simulink model "BGOnly_5CH"  (R2017b)
settings: Solver=VariableStepAuto  StartTime=0.0  StopTime=60  RelTol=1e-3  EnableMultiTasking=on
values from neighbouring files (symbols this model uses):
  CHNoise = 1e-05    [Extension 1 Variables.mat]    (also in PlotChannelDiscrete.m = 1e-10; PlotChannelsExt.m = 0.0001; SelectivityFunction.m = 0.001)
  teta = 0.02    [Extension 1 Variables.mat]
  w_e = 0.9    [Extension 1 Variables.mat]    (also in PlotChannelsExt.m = 1)
  w_g = 1    [Extension 1 Variables.mat]
  w_minus = 1    [Extension 1 Variables.mat]    (also in PlotChannelsExt.m = 1.05)
  w_plus = 0.9    [Extension 1 Variables.mat]    (also in PlotChannelsExt.m = 1)
  w_s = 1    [Extension 1 Variables.mat]    (also in PlotChannelsExt.m)
  w_t = 0.9    [Extension 1 Variables.mat]    (also in PlotChannelsExt.m = 1)
undefined symbols (not defined in the file or in its folder): sigbuilder_block
libraries: fuzblock x25, simulink x8
settings Model: Creator=User  LastModifiedBy=acaso
settings DataIOCC: LimitDataPoints=on
settings OptimizationCC: LifeSpan=inf
settings DebuggingCC: AllowSymbolicDim=off  SFUnexpectedBacktrackingDiag=warning  SFNoUnconditionalDefaultTransitionDiag=warning  SFExecutionAtInitializationDiag=none
settings ModelReferenceCC: PropagateSignalLabelsOutOfModel=off
settings CodeAppCC: StateflowObjectComments=on
settings GRTTargetCC: TargetLangStandard=C89/C90 (ANSI)
settings ConfigComp: CovMetricSettings=dw  CovHtmlReporting=on  CovSaveCumulativeToWorkspaceVar=on  CovSaveSingleToWorkspaceVar=on  CovExternalEMLEnable=off

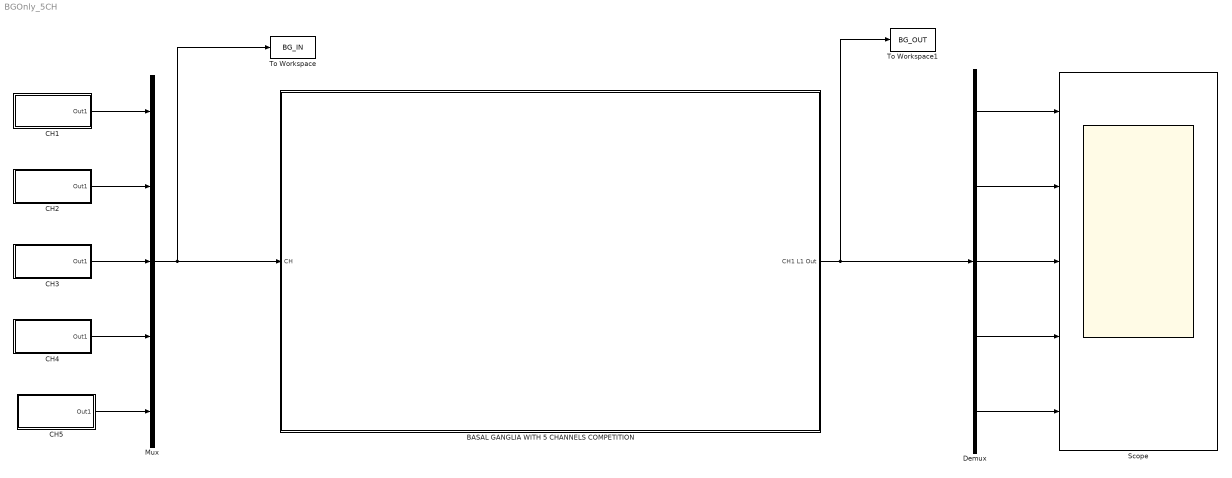
== system BGOnly_5CH ==
  BASAL GANGLIA WITH 5 CHANNELS COMPETITION : Subsystem
  "CH1 " : Subsystem
  CH2 : Subsystem
  "CH3 " : Subsystem
  "CH4 " : Subsystem
  "CH5 " : Subsystem
  Demux : Demux  Outputs=5
  Mux : Mux  Inputs=5
  Scope : Scope  NumInputPorts=5
  To Workspace : ToWorkspace  VariableName=BG_IN  SaveFormat=Timeseries  SampleTime=0.1
  To Workspace1 : ToWorkspace  VariableName=BG_OUT  SaveFormat=Timeseries  SampleTime=0.1
  wires:
  Mux/1 -> To Workspace/1, BASAL GANGLIA WITH 5 CHANNELS COMPETITION/1("CH ")
  BASAL GANGLIA WITH 5 CHANNELS COMPETITION/1(CH1 L1 Out) -> To Workspace1/1, Demux/1
  Demux/5 -> Scope/5
  Demux/4 -> Scope/4
  Demux/3 -> Scope/3
  Demux/2 -> Scope/2
  Demux/1 -> Scope/1
  "CH1 "/1(Out1) -> Mux/1
  CH2/1(Out1) -> Mux/2
  "CH3 "/1(Out1) -> Mux/3
  "CH4 "/1(Out1) -> Mux/4
  "CH5 "/1(Out1) -> Mux/5

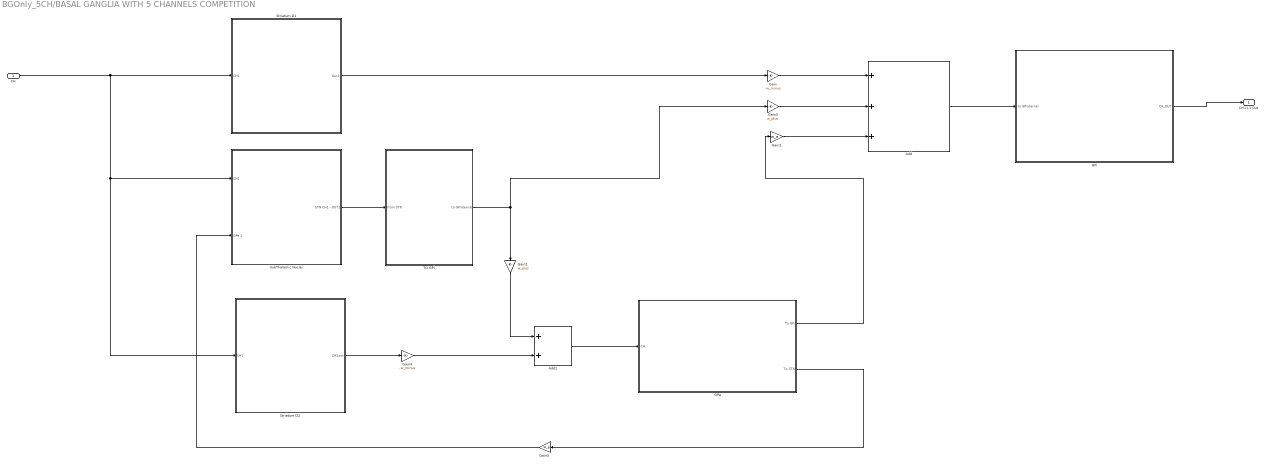
== system BGOnly_5CH/BASAL GANGLIA WITH 5 CHANNELS COMPETITION ==
  "CH " : Inport
  Add : Sum  Inputs=3
  Add1 : Sum  Inputs=2
  GPe : Subsystem  TreatAsAtomicUnit=on
  GPi : Subsystem
  Gain : Gain  Gain=-w_minus
  Gain1 : Gain  Gain=w_e
  Gain2 : Gain  Gain=w_plus
  Gain3 : Gain  Gain=w_plus
  Gain4 : Gain  Gain=-w_minus
  Gain5 : Gain  Gain=-w_g
  "Striatum D1 " : Subsystem
  Striatum D2 : Subsystem
  SubThalamic Nuclei : Subsystem
  TO GPi : Subsystem
  CH1 L1 Out : Outport
  wires:
  TO GPi/1(to GPinternal) -> Gain3/1, Gain2/1
  GPi/1("CH_OUT ") -> CH1 L1 Out/1
  "CH "/1 -> Striatum D2/1(CH1), SubThalamic Nuclei/1(CH1), "Striatum D1 "/1(CH1)
  "Striatum D1 "/1(Out1) -> Gain/1
  SubThalamic Nuclei/1(STN CH1 - OUT1) -> TO GPi/1("from STN ")
  GPe/1(To GPi) -> Gain1/1
  Gain/1 -> Add/1
  Gain3/1 -> Add/2
  Gain1/1 -> Add/3
  Striatum D2/1(CH1out) -> Gain4/1
  Gain2/1 -> Add1/1
  Gain4/1 -> Add1/2
  Add1/1 -> GPe/1(CH)
  GPe/2(To STN) -> Gain5/1
  Gain5/1 -> SubThalamic Nuclei/2(GPe 1)
  Add/1 -> GPi/1("to GPinternal ")

== system BGOnly_5CH/CH1  ==
  Add : Sum
  Band-Limited White Noise : simulink/Sources/Band-Limited White Noise  Cov=[CHNoise]  Ts=0.1  seed=[23341]
  "CHANNEL1 IN " : Subsystem  Tag=STV Subsys  LoadFcn=sigbuilder_block('load');  StartFcn=sigbuilder_block('start');  StopFcn=sigbuilder_block('stop');  ClipboardFcn=sigbuilder_block('clipboard');  mask(Sigbuilder block){tuvar=[0:10]}
      mask help: Simulink:masks:SigbuilderBlock_MD
      mask init:
      | if ~strcmp(get_param(bdroot(gcbh),'SimulationStatus'),'stopped') tuvar = sigbuilder_block('maskInit'); end
      settings: CopyFcn=sigbuilder_block('copy');  DeleteFcn=sigbuilder_block('delete');  ModelCloseFcn=sigbuilder_block('modelClose');  PreSaveFcn=sigbuilder_block('preSave');  PauseFcn=sigbuilder_block('pause');  ContinueFcn=sigbuilder_block('continue');  NameChangeFcn=sigbuilder_block('namechange');  OpenFcn=sigbuilder_block('open',[5.4 5.4 1141.2 580.8 ]);  CloseFcn=sigbuilder_block('close');
      mask Display: plot(0, 0, 100, 100,[2, 2, 32, 32, 2], [68, 8, 8, 68, 68],[32, 2], [38, 38], [32, 19, 2],[53, 60, 44], [32, 17, 17, 2],[16, 16, 31, 31]);txt = getActiveGroup(gcbh);text(2, 100, txt,'verticalAlignment', 'top');
  Out1 : Outport
  wires:
  Band-Limited White Noise/1 -> Add/2
  Add/1 -> Out1/1
  "CHANNEL1 IN "/1(Signal 1) -> Add/1

== system BGOnly_5CH/CH2 ==
  Add : Sum
  Band-Limited White Noise : simulink/Sources/Band-Limited White Noise  Cov=[CHNoise]  Ts=0.1  seed=[23341]
  "CHANNEL2 IN " : Subsystem  Tag=STV Subsys  LoadFcn=sigbuilder_block('load');  StartFcn=sigbuilder_block('start');  StopFcn=sigbuilder_block('stop');  ClipboardFcn=sigbuilder_block('clipboard');  mask(Sigbuilder block){tuvar=[0:10]}
      mask help: Simulink:masks:SigbuilderBlock_MD
      mask init:
      | if ~strcmp(get_param(bdroot(gcbh),'SimulationStatus'),'stopped') tuvar = sigbuilder_block('maskInit'); end
      settings: CopyFcn=sigbuilder_block('copy');  DeleteFcn=sigbuilder_block('delete');  ModelCloseFcn=sigbuilder_block('modelClose');  PreSaveFcn=sigbuilder_block('preSave');  PauseFcn=sigbuilder_block('pause');  ContinueFcn=sigbuilder_block('continue');  NameChangeFcn=sigbuilder_block('namechange');  OpenFcn=sigbuilder_block('open',[161.4 5.4 877.8 580.8 ]);  CloseFcn=sigbuilder_block('close');
      mask Display: plot(0, 0, 100, 100,[2, 2, 32, 32, 2], [68, 8, 8, 68, 68],[32, 2], [38, 38], [32, 19, 2],[53, 60, 44], [32, 17, 17, 2],[16, 16, 31, 31]);txt = getActiveGroup(gcbh);text(2, 100, txt,'verticalAlignment', 'top');
  Out1 : Outport
  wires:
  Band-Limited White Noise/1 -> Add/2
  Add/1 -> Out1/1
  "CHANNEL2 IN "/3(Signal 3) -> Add/1

== system BGOnly_5CH/CH3  ==
  Add : Sum
  Band-Limited White Noise : simulink/Sources/Band-Limited White Noise  Cov=[CHNoise]  Ts=0.1  seed=[23341]
  "CHANNEL2 IN " : Subsystem  Tag=STV Subsys  LoadFcn=sigbuilder_block('load');  StartFcn=sigbuilder_block('start');  StopFcn=sigbuilder_block('stop');  ClipboardFcn=sigbuilder_block('clipboard');  mask(Sigbuilder block){tuvar=[0:10]}
      mask help: Simulink:masks:SigbuilderBlock_MD
      mask init:
      | if ~strcmp(get_param(bdroot(gcbh),'SimulationStatus'),'stopped') tuvar = sigbuilder_block('maskInit'); end
      settings: CopyFcn=sigbuilder_block('copy');  DeleteFcn=sigbuilder_block('delete');  ModelCloseFcn=sigbuilder_block('modelClose');  PreSaveFcn=sigbuilder_block('preSave');  PauseFcn=sigbuilder_block('pause');  ContinueFcn=sigbuilder_block('continue');  NameChangeFcn=sigbuilder_block('namechange');  OpenFcn=sigbuilder_block('open',[5.4 5.4 1141.2 580.8 ]);  CloseFcn=sigbuilder_block('close');
      mask Display: plot(0, 0, 100, 100,[2, 2, 32, 32, 2], [68, 8, 8, 68, 68],[32, 2], [38, 38], [32, 19, 2],[53, 60, 44], [32, 17, 17, 2],[16, 16, 31, 31]);txt = getActiveGroup(gcbh);text(2, 100, txt,'verticalAlignment', 'top');
  Out1 : Outport
  wires:
  Band-Limited White Noise/1 -> Add/2
  Add/1 -> Out1/1
  "CHANNEL2 IN "/1(Signal 3) -> Add/1

== system BGOnly_5CH/CH4  ==
  Add : Sum
  Band-Limited White Noise : simulink/Sources/Band-Limited White Noise  Cov=[CHNoise]  Ts=0.1  seed=[23341]
  "CHANNEL2 IN " : Subsystem  Tag=STV Subsys  LoadFcn=sigbuilder_block('load');  StartFcn=sigbuilder_block('start');  StopFcn=sigbuilder_block('stop');  ClipboardFcn=sigbuilder_block('clipboard');  mask(Sigbuilder block){tuvar=[0:10]}
      mask help: Simulink:masks:SigbuilderBlock_MD
      mask init:
      | if ~strcmp(get_param(bdroot(gcbh),'SimulationStatus'),'stopped') tuvar = sigbuilder_block('maskInit'); end
      settings: CopyFcn=sigbuilder_block('copy');  DeleteFcn=sigbuilder_block('delete');  ModelCloseFcn=sigbuilder_block('modelClose');  PreSaveFcn=sigbuilder_block('preSave');  PauseFcn=sigbuilder_block('pause');  ContinueFcn=sigbuilder_block('continue');  NameChangeFcn=sigbuilder_block('namechange');  OpenFcn=sigbuilder_block('open',[5.4 5.4 1141.2 580.8 ]);  CloseFcn=sigbuilder_block('close');
      mask Display: plot(0, 0, 100, 100,[2, 2, 32, 32, 2], [68, 8, 8, 68, 68],[32, 2], [38, 38], [32, 19, 2],[53, 60, 44], [32, 17, 17, 2],[16, 16, 31, 31]);txt = getActiveGroup(gcbh);text(2, 100, txt,'verticalAlignment', 'top');
  Out1 : Outport
  wires:
  Band-Limited White Noise/1 -> Add/2
  Add/1 -> Out1/1
  "CHANNEL2 IN "/1(Signal 3) -> Add/1

== system BGOnly_5CH/CH5  ==
  Add : Sum
  Band-Limited White Noise : simulink/Sources/Band-Limited White Noise  Cov=[CHNoise]  Ts=0.1  seed=[23341]
  "CHANNEL2 IN " : Subsystem  Tag=STV Subsys  LoadFcn=sigbuilder_block('load');  StartFcn=sigbuilder_block('start');  StopFcn=sigbuilder_block('stop');  ClipboardFcn=sigbuilder_block('clipboard');  mask(Sigbuilder block){tuvar=[0:10]}
      mask help: Simulink:masks:SigbuilderBlock_MD
      mask init:
      | if ~strcmp(get_param(bdroot(gcbh),'SimulationStatus'),'stopped') tuvar = sigbuilder_block('maskInit'); end
      settings: CopyFcn=sigbuilder_block('copy');  DeleteFcn=sigbuilder_block('delete');  ModelCloseFcn=sigbuilder_block('modelClose');  PreSaveFcn=sigbuilder_block('preSave');  PauseFcn=sigbuilder_block('pause');  ContinueFcn=sigbuilder_block('continue');  NameChangeFcn=sigbuilder_block('namechange');  OpenFcn=sigbuilder_block('open',[5.4 5.4 1141.2 580.8 ]);  CloseFcn=sigbuilder_block('close');
      mask Display: plot(0, 0, 100, 100,[2, 2, 32, 32, 2], [68, 8, 8, 68, 68],[32, 2], [38, 38], [32, 19, 2],[53, 60, 44], [32, 17, 17, 2],[16, 16, 31, 31]);txt = getActiveGroup(gcbh);text(2, 100, txt,'verticalAlignment', 'top');
  Out1 : Outport
  wires:
  Band-Limited White Noise/1 -> Add/2
  Add/1 -> Out1/1
  "CHANNEL2 IN "/1(Signal 3) -> Add/1

== system BGOnly_5CH/BASAL GANGLIA WITH 5 CHANNELS COMPETITION/GPe ==
  CH : Inport
  GPe CH1 : Subsystem
  To GPi : Outport
  To STN : Outport  Port=2
  wires:
  CH/1 -> GPe CH1/1(In)
  GPe CH1/1(To GPi) -> To GPi/1
  GPe CH1/2(To STN) -> To STN/1

== system BGOnly_5CH/BASAL GANGLIA WITH 5 CHANNELS COMPETITION/GPi ==
  "to GPinternal " : Inport
  GPinternal : Subsystem
  "CH_OUT " : Outport
  wires:
  "to GPinternal "/1 -> GPinternal/1("to GPinternal ")
  GPinternal/1(To Thal) -> "CH_OUT "/1

== system BGOnly_5CH/BASAL GANGLIA WITH 5 CHANNELS COMPETITION/Striatum D1  ==
  CH1 : Inport
  "Striatum D1 " : Subsystem
  Out1 : Outport
  wires:
  CH1/1 -> "Striatum D1 "/1(Channel)
  "Striatum D1 "/1(Striatum D1 Out) -> Out1/1

== system BGOnly_5CH/BASAL GANGLIA WITH 5 CHANNELS COMPETITION/Striatum D2 ==
  CH1 : Inport
  Scope : Scope
  "Striatum D2 " : Subsystem
  CH1out : Outport
  wires:
  "Striatum D2 "/1(Striatum D1 Out) -> Scope/1, CH1out/1
  CH1/1 -> "Striatum D2 "/1(Channel)

== system BGOnly_5CH/BASAL GANGLIA WITH 5 CHANNELS COMPETITION/SubThalamic Nuclei ==
  CH1 : Inport
  GPe 1 : Inport  Port=2
  "SubThalamic Nucleus (STN) " : Subsystem
  STN CH1 - OUT1 : Outport
  wires:
  CH1/1 -> "SubThalamic Nucleus (STN) "/1(Channel)
  GPe 1/1 -> "SubThalamic Nucleus (STN) "/2(GPe Inp)
  "SubThalamic Nucleus (STN) "/1(STN Out1) -> STN CH1 - OUT1/1

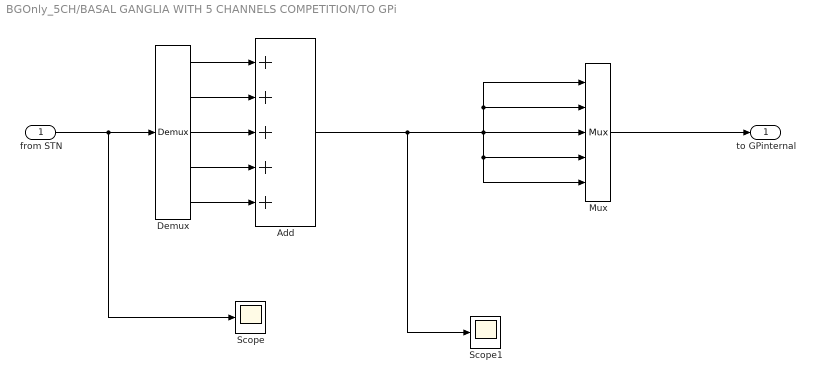
== system BGOnly_5CH/BASAL GANGLIA WITH 5 CHANNELS COMPETITION/TO GPi ==
  "from STN " : Inport
  Add : Sum  Inputs=5
  Demux : Demux  Outputs=5
  Mux : Mux  Inputs=5
  Scope : Scope
  Scope1 : Scope
  to GPinternal : Outport
  wires:
  "from STN "/1 -> Scope/1, Demux/1
  Demux/1 -> Add/1
  Demux/2 -> Add/2
  Demux/3 -> Add/3
  Demux/4 -> Add/4
  Demux/5 -> Add/5
  Add/1 -> Scope1/1, Mux/1, Mux/2, Mux/3, Mux/4, Mux/5
  Mux/1 -> to GPinternal/1

== system BGOnly_5CH/CH1 /CHANNEL1 IN  ==
  Demux : Demux  Tag=STV Demux  Outputs=2
  FromWs : FromWorkspace  Tag=STV FromWs  VariableName=tuvar  SampleTime=0
      SigBuilderData=|
      | common.afterFinalStr = 'Extrapolate'
      | common.sampleTime = 0
      | dataSet.timeRange = [0 35]
      | dataSet.name = 'Group 1'
      | sbobj.Groups.Name = 'Group 1'
      | sbobj.Groups.Signals(1).Name = 'Signal 1'
      | sbobj.Groups.Signals(1).XData = [0 0.125 0.25 0.375 0.5 0.625 0.75 0.875 1 1.125 1.25 1.375 1.5 1.625 1.75 1.875 2 2.125 2.25 2.375 2.5 2.625 2.75 2.875 3 3.125 3.25 3.375 3.5 3.625 3.75 3.875 4 4.125 4.25 4.375 4.5 4.625 4.75 4.875 5 5.125 5.25 5.375 5.5 5.625 5.75 5.875 6 6.125 6.25 6.375 6.5 6.625 6.75 6.875 7 7.125 7.25 7.375 7.5 7.625 7.75 7.875 8 8.125 8.25 8.375 8.5 8.625 8.75 8.875 9 9.125 9.25 9.375 9.5 9.625 9.75 9.875 10 10.125 10.25 10.375 10.5 10.625 10.75 10.875 11 11.125 11.25 11.375 11.5 11.625 11.75 11.875 12 12.125 12.25 12.375 12.5 12.625 12.75 12.875 13 13.125 13.25 13.375 13.5 13.625 13.75 13.875 14 14.125 14.25 14.375 14.5 14.625 14.75 14.875 15 15.125 15.25 15.375 15.5 15.625 15.75 15.875 16 16.125 16.25 16.375 16.5 16.625 16.75 16.875 17 17.125 17.25 17.375 17.5 17.625 17.75 17.875 18 18.125 18.25 18.375 18.5 18.625 18.75 18.875 19 19.125 19.25 19.375 19.5 19.625 19.75 19.875 20 20.125 20.25 20.375 20.5 20.625 20.75 20.875 21 21.125 21.25 21.375 21.5 21.625 21.75 21.875 22 22.125 22.25 22.375 22.5 22.625 22.75 22.875 23 23.125 23.25 23.375 23.5 23.625 23.75 23.875 24 24.125 24.25 24.375 24.5 24.625 24.75 24.875 25 25.125 25.25 25.375 25.5 25.625 25.75 25.875 26 26.125 26.25 26.375 26.5 26.625 26.75 26.875 27 27.125 27.25 27.375 27.5 27.625 27.75 27.875 28 28.125 28.25 28.375 28.5 28.625 28.75 28.875 29 29.125 29.25 29.375 29.5 29.625 29.75 29.875 30 30.125 30.25 30.375 30.5 30.625 30.75 30.875 31 31.125 31.25 31.375 31.5 31.625 31.75 31.875 32 32.125 32.25 32.375 32.5 32.625 32.75 32.875 33 33.125 33.25 33.375 33.5 33.625 33.75 33.875 34 34.125 34.25 34.375 34.5 34.625 34.75 34.875 35]
      | sbobj.Groups.Signals(1).YData = [1 1.70710678119 2 1.70710678119 1 0.292893218813 0 0.292893218813 1 1.70710678119 2 1.70710678119 ... (281 elements, 1x281)]
      | sbobj.Groups.Signals(2).Name = 'Signal 2'
      | sbobj.Groups.Signals(2).XData = [0 10 10 19.95 19.95 35]
      | sbobj.Groups.Signals(2).YData = [0 0 1 1 0 0]
      | sbobj.Groups.TimeRange = [0 35]
  Signal 1 : Outport  Tag=STV Outport
  Signal 2 : Outport  Tag=STV Outport  Port=2
  wires:
  Demux/1 -> Signal 1/1
  FromWs/1 -> Demux/1
  Demux/2 -> Signal 2/1

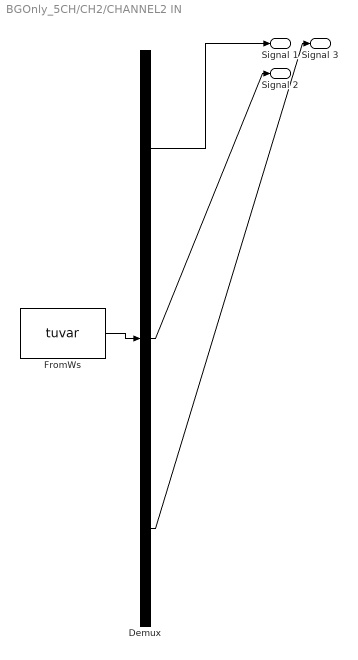
== system BGOnly_5CH/CH2/CHANNEL2 IN  ==
  Demux : Demux  Tag=STV Demux  Outputs=3
  FromWs : FromWorkspace  Tag=STV FromWs  VariableName=tuvar  SampleTime=0
      SigBuilderData=|
      | common.afterFinalStr = 'Extrapolate'
      | common.sampleTime = 0
      | dataSet.timeRange = [0 35]
      | dataSet.name = 'Group 1'
      | sbobj.Groups.Name = 'Group 1'
      | sbobj.Groups.Signals(1).Name = 'Signal 1'
      | sbobj.Groups.Signals(1).XData = [0 10 10 15.05 15.05 20 20 24.95 24.95 30 30 35]
      | sbobj.Groups.Signals(1).YData = [-0.002 -0.002 0.40108 0.402 0.598 0.598 0.898 0.898 0.405 0.405 -0.002 -0.002]
      | sbobj.Groups.Signals(2).Name = 'Signal 2'
      | sbobj.Groups.Signals(2).XData = [0 15 15 25.05 25.05 35]
      | sbobj.Groups.Signals(2).YData = [0 0 1 1 0 0]
      | sbobj.Groups.Signals(3).Name = 'Signal 3'
      | sbobj.Groups.Signals(3).XData = [0 0.25 0.5 0.75 1 1.25 1.5 1.75 2 2.25 2.5 2.75 3 3.25 3.5 3.75 4 4.25 4.5 4.75 5 5.25 5.5 5.75 6 6.25 6.5 6.75 7 7.25 7.5 7.75 8 8.25 8.5 8.75 9 9.25 9.5 9.75 10 10.25 10.5 10.75 11 11.25 11.5 11.75 12 12.25 12.5 12.75 13 13.25 13.5 13.75 14 14.25 14.5 14.75 15 15.25 15.5 15.75 16 16.25 16.5 16.75 17 17.25 17.5 17.75 18 18.25 18.5 18.75 19 19.25 19.5 19.75 20 20.25 20.5 20.75 21 21.25 21.5 21.75 22 22.25 22.5 22.75 23 23.25 23.5 23.75 24 24.25 24.5 24.75 25 25.25 25.5 25.75 26 26.25 26.5 26.75 27 27.25 27.5 27.75 28 28.25 28.5 28.75 29 29.25 29.5 29.75 30 30.25 30.5 30.75 31 31.25 31.5 31.75 32 32.25 32.5 32.75 33 33.25 33.5 33.75 34 34.25 34.5 34.75 35]
      | sbobj.Groups.Signals(3).YData = [1 1.70710678119 2 1.70710678119 1 0.292893218813 0 0.292893218813 1 1.70710678119 2 1.70710678119 1 0.292893218813 0 0.292893218813 1 1.70710678119 2 1.70710678119 1 0.292893218813 0 0.292893218813 1 1.70710678119 2 1.70710678119 1 0.292893218813 0 0.292893218813 1 1.70710678119 2 1.70710678119 1 0.292893218813 0 0.292893218813 1 1.70710678119 2 1.70710678119 1 0.292893218813 0 0.292893218813 1 1.70710678119 2 1.70710678119 1 0.292893218813 0 0.292893218813 1 1.70710678119 2 1.70710678119 1 0.292893218813 0 0.292893218813 1 1.70710678119 2 1.70710678119 1 0.292893218813 0 0.292893218813 1 1.70710678119 2 1.70710678119 1 0.292893218813 0 0.292893218813 1 1.70710678119 2 1.70710678119 1 0.292893218813 0 0.292893218813 1 1.70710678119 2 1.70710678119 1 0.292893218813 0 0.292893218813 1 1.70710678119 2 1.70710678119 1 0.292893218813 0 0.292893218813 1 1.70710678119 2 1.70710678119 1 0.292893218813 0 0.292893218813 1 1.70710678119 2 1.70710678119 1 0.292893218813 0 0.292893218813 1 1.70710678119 2 1.70710678119 1 0.292893218813 0 0.292893218813 1 1.70710678119 2 1.70710678119 1 0.292893218813 0 0.292893218813 1 1.70710678119 2 1.70710678119 1]
      | sbobj.Groups.TimeRange = [0 35]
  Signal 1 : Outport  Tag=STV Outport
  Signal 2 : Outport  Tag=STV Outport  Port=2
  Signal 3 : Outport  Tag=STV Outport  Port=3
  wires:
  Demux/1 -> Signal 1/1
  FromWs/1 -> Demux/1
  Demux/2 -> Signal 2/1
  Demux/3 -> Signal 3/1

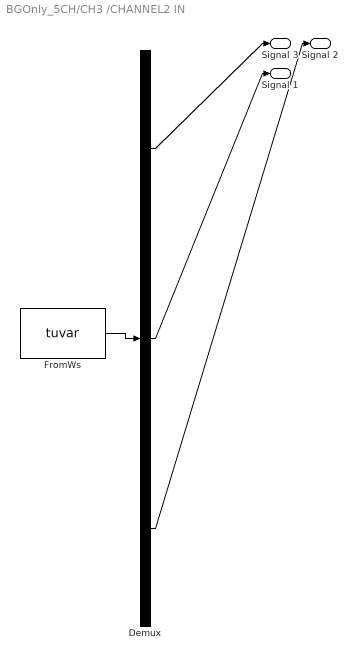
== system BGOnly_5CH/CH3 /CHANNEL2 IN  ==
  Demux : Demux  Tag=STV Demux  Outputs=3
  FromWs : FromWorkspace  Tag=STV FromWs  VariableName=tuvar  SampleTime=0
      SigBuilderData=|
      | common.afterFinalStr = 'Extrapolate'
      | common.sampleTime = 0
      | dataSet.timeRange = [0 35]
      | dataSet.name = 'Group 1'
      | sbobj.Groups.Name = 'Group 1'
      | sbobj.Groups.Signals(1).Name = 'Signal 3'
      | sbobj.Groups.Signals(1).XData = [0 35]
      | sbobj.Groups.Signals(1).YData = [0.195 0.195]
      | sbobj.Groups.Signals(2).Name = 'Signal 1'
      | sbobj.Groups.Signals(2).XData = [0 25 25 32.85 32.85 35]
      | sbobj.Groups.Signals(2).YData = [0 0 1 1 0 0]
      | sbobj.Groups.Signals(3).Name = 'Signal 2'
      | sbobj.Groups.Signals(3).XData = [0 0.5 1 1.5 2 2.5 3 3.5 4 4.5 5 5.5 6 6.5 7 7.5 8 8.5 9 9.5 10 10.5 11 11.5 12 12.5 13 13.5 14 14.5 15 15.5 16 16.5 17 17.5 18 18.5 19 19.5 20 20.5 21 21.5 22 22.5 23 23.5 24 24.5 25 25.5 26 26.5 27 27.5 28 28.5 29 29.5 30 30.5 31 31.5 32 32.5 33 33.5 34 34.5 35]
      | sbobj.Groups.Signals(3).YData = [1 1.70710678119 2 1.70710678119 1 0.292893218813 0 0.292893218813 1 1.70710678119 2 1.70710678119 1 0.292893218813 0 0.292893218813 1 1.70710678119 2 1.70710678119 1 0.292893218813 0 0.292893218813 1 1.70710678119 2 1.70710678119 1 0.292893218813 0 0.292893218813 1 1.70710678119 2 1.70710678119 1 0.292893218813 0 0.292893218813 1 1.70710678119 2 1.70710678119 1 0.292893218813 0 0.292893218813 1 1.70710678119 2 1.70710678119 1 0.292893218813 0 0.292893218813 1 1.70710678119 2 1.70710678119 1 0.292893218813 0 0.292893218813 1 1.70710678119 2 1.70710678119 1 0.292893218813 0]
      | sbobj.Groups.TimeRange = [0 35]
  Signal 3 : Outport  Tag=STV Outport
  Signal 1 : Outport  Tag=STV Outport  Port=2
  Signal 2 : Outport  Tag=STV Outport  Port=3
  wires:
  FromWs/1 -> Demux/1
  Demux/1 -> Signal 3/1
  Demux/2 -> Signal 1/1
  Demux/3 -> Signal 2/1

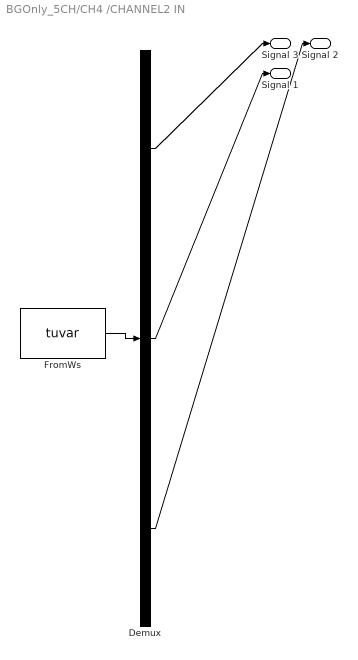
== system BGOnly_5CH/CH4 /CHANNEL2 IN  ==
  Demux : Demux  Tag=STV Demux  Outputs=3
  FromWs : FromWorkspace  Tag=STV FromWs  VariableName=tuvar  SampleTime=0
      SigBuilderData=|
      | common.afterFinalStr = 'Extrapolate'
      | common.sampleTime = 0
      | dataSet.timeRange = [0 35]
      | dataSet.name = 'Group 1'
      | sbobj.Groups.Name = 'Group 1'
      | sbobj.Groups.Signals(1).Name = 'Signal 3'
      | sbobj.Groups.Signals(1).XData = [0 35]
      | sbobj.Groups.Signals(1).YData = [0.12 0.12]
      | sbobj.Groups.Signals(2).Name = 'Signal 1'
      | sbobj.Groups.Signals(2).XData = [0 28.15 28.15 31.75 31.75 35]
      | sbobj.Groups.Signals(2).YData = [0 0 1 1 0 0]
      | sbobj.Groups.Signals(3).Name = 'Signal 2'
      | sbobj.Groups.Signals(3).XData = [0 1 2 3 4 5 6 7 8 9 10 11 12 13 14 15 16 17 18 19 20 21 22 23 24 25 26 27 28 29 30 31 32 33 34 35]
      | sbobj.Groups.Signals(3).YData = [1 1.70710678119 2 1.70710678119 1 0.292893218813 0 0.292893218813 1 1.70710678119 2 1.70710678119 1 0.292893218813 0 0.292893218813 1 1.70710678119 2 1.70710678119 1 0.292893218813 0 0.292893218813 1 1.70710678119 2 1.70710678119 1 0.292893218813 0 0.292893218813 1 1.70710678119 2 1.70710678119]
      | sbobj.Groups.TimeRange = [0 35]
  Signal 3 : Outport  Tag=STV Outport
  Signal 1 : Outport  Tag=STV Outport  Port=2
  Signal 2 : Outport  Tag=STV Outport  Port=3
  wires:
  FromWs/1 -> Demux/1
  Demux/1 -> Signal 3/1
  Demux/2 -> Signal 1/1
  Demux/3 -> Signal 2/1

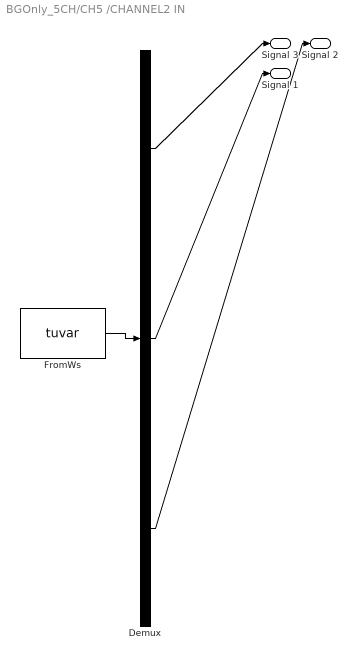
== system BGOnly_5CH/CH5 /CHANNEL2 IN  ==
  Demux : Demux  Tag=STV Demux  Outputs=3
  FromWs : FromWorkspace  Tag=STV FromWs  VariableName=tuvar  SampleTime=0
      SigBuilderData=|
      | common.afterFinalStr = 'Extrapolate'
      | common.sampleTime = 0
      | dataSet.timeRange = [0 35]
      | dataSet.name = 'Group 1'
      | sbobj.Groups.Name = 'Group 1'
      | sbobj.Groups.Signals(1).Name = 'Signal 3'
      | sbobj.Groups.Signals(1).XData = [0 35]
      | sbobj.Groups.Signals(1).YData = [0.085 0.085]
      | sbobj.Groups.Signals(2).Name = 'Signal 1'
      | sbobj.Groups.Signals(2).XData = [0 29.7 29.7 33.95 33.95 35]
      | sbobj.Groups.Signals(2).YData = [0.051 0.051 0.78 0.78 0.049 0.049]
      | sbobj.Groups.Signals(3).Name = 'Signal 2'
      | sbobj.Groups.Signals(3).XData = [0 2 4 6 8 10 12 14 16 18 20 22 24 26 28 30 32 34 35]
      | sbobj.Groups.Signals(3).YData = [1 1.70710678119 2 1.70710678119 1 0.292893218813 0 0.292893218813 1 1.70710678119 2 1.70710678119 1 0.292893218813 0 0.292893218813 1 1.70710678119 1.92387953251]
      | sbobj.Groups.TimeRange = [0 35]
  Signal 3 : Outport  Tag=STV Outport
  Signal 1 : Outport  Tag=STV Outport  Port=2
  Signal 2 : Outport  Tag=STV Outport  Port=3
  wires:
  FromWs/1 -> Demux/1
  Demux/1 -> Signal 3/1
  Demux/2 -> Signal 1/1
  Demux/3 -> Signal 2/1

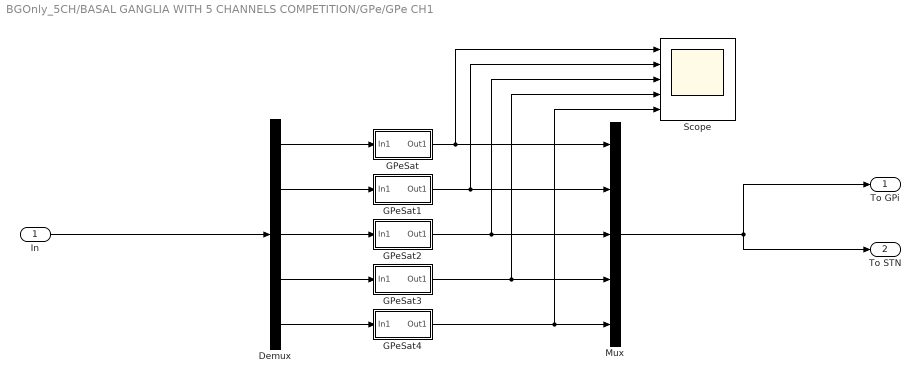
== system BGOnly_5CH/BASAL GANGLIA WITH 5 CHANNELS COMPETITION/GPe/GPe CH1 ==
  In : Inport
  Demux : Demux  Outputs=5
  GPeSat : Subsystem
  GPeSat1 : Subsystem
  GPeSat2 : Subsystem
  GPeSat3 : Subsystem
  GPeSat4 : Subsystem
  Mux : Mux  Inputs=5
  Scope : Scope  NumInputPorts=5
  To GPi : Outport
  To STN : Outport  Port=2
  wires:
  Mux/1 -> To STN/1, To GPi/1
  Demux/1 -> GPeSat/1(In1)
  GPeSat/1(Out1) -> Scope/1, Mux/1
  Demux/2 -> GPeSat1/1(In1)
  GPeSat1/1(Out1) -> Scope/2, Mux/2
  Demux/3 -> GPeSat2/1(In1)
  GPeSat2/1(Out1) -> Scope/3, Mux/3
  Demux/4 -> GPeSat3/1(In1)
  GPeSat3/1(Out1) -> Scope/4, Mux/4
  Demux/5 -> GPeSat4/1(In1)
  GPeSat4/1(Out1) -> Scope/5, Mux/5
  In/1 -> Demux/1

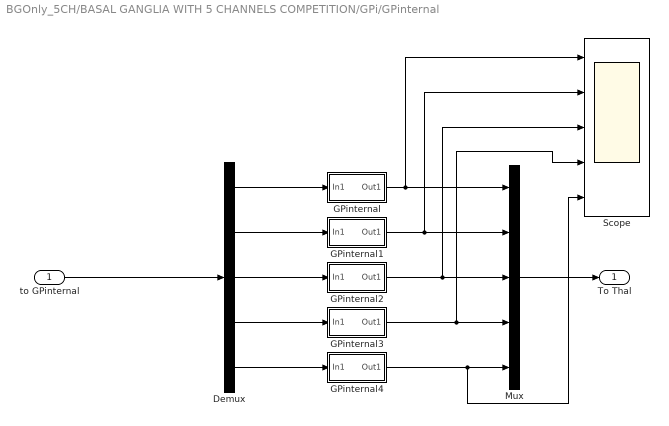
== system BGOnly_5CH/BASAL GANGLIA WITH 5 CHANNELS COMPETITION/GPi/GPinternal ==
  "to GPinternal " : Inport
  Demux : Demux  Outputs=5
  GPinternal : Subsystem
  GPinternal1 : Subsystem
  GPinternal2 : Subsystem
  GPinternal3 : Subsystem
  GPinternal4 : Subsystem
  Mux : Mux  Inputs=5
  Scope : Scope  NumInputPorts=5
  To Thal : Outport
  wires:
  Demux/1 -> GPinternal/1(In1)
  GPinternal/1(Out1) -> Mux/1, Scope/1
  Demux/2 -> GPinternal1/1(In1)
  Demux/3 -> GPinternal2/1(In1)
  GPinternal2/1(Out1) -> Scope/3, Mux/3
  Demux/4 -> GPinternal3/1(In1)
  GPinternal3/1(Out1) -> Scope/4, Mux/4
  Demux/5 -> GPinternal4/1(In1)
  GPinternal4/1(Out1) -> Scope/5, Mux/5
  Mux/1 -> To Thal/1
  GPinternal1/1(Out1) -> Scope/2, Mux/2
  "to GPinternal "/1 -> Demux/1

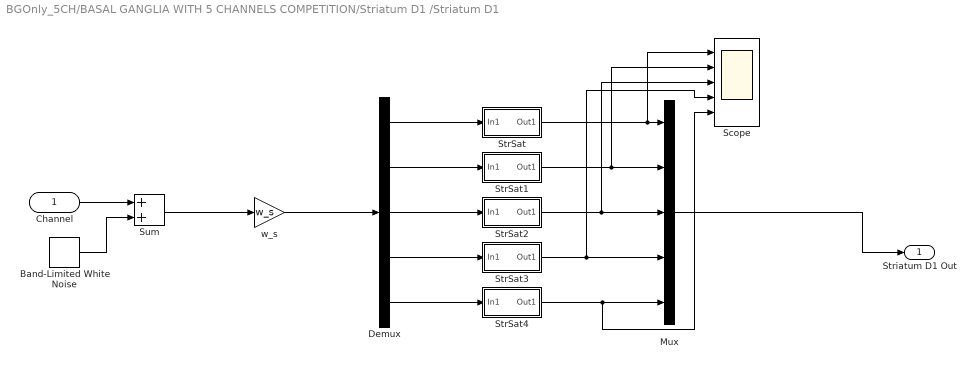
== system BGOnly_5CH/BASAL GANGLIA WITH 5 CHANNELS COMPETITION/Striatum D1 /Striatum D1  ==
  Channel : Inport
  Band-Limited White Noise : simulink/Sources/Band-Limited White Noise  Cov=[0]  Ts=0.1  seed=[23341]
  Demux : Demux  Outputs=5
  Mux : Mux  Inputs=5
  Scope : Scope  NumInputPorts=5
  StrSat : Subsystem
  StrSat1 : Subsystem
  StrSat2 : Subsystem
  StrSat3 : Subsystem
  StrSat4 : Subsystem
  Sum : Sum
  w_s : Gain  Gain=w_s
  Striatum D1 Out : Outport
  wires:
  Channel/1 -> Sum/1
  Sum/1 -> w_s/1
  Mux/1 -> Striatum D1 Out/1
  Band-Limited White Noise/1 -> Sum/2
  Demux/1 -> StrSat/1(In1)
  StrSat/1(Out1) -> Scope/1, Mux/1
  Demux/2 -> StrSat1/1(In1)
  StrSat1/1(Out1) -> Scope/2, Mux/2
  Demux/3 -> StrSat2/1(In1)
  StrSat2/1(Out1) -> Scope/3, Mux/3
  Demux/4 -> StrSat3/1(In1)
  StrSat3/1(Out1) -> Scope/4, Mux/4
  Demux/5 -> StrSat4/1(In1)
  StrSat4/1(Out1) -> Scope/5, Mux/5
  w_s/1 -> Demux/1

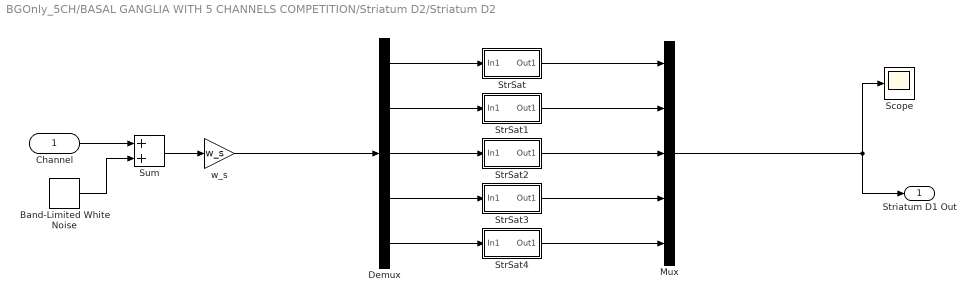
== system BGOnly_5CH/BASAL GANGLIA WITH 5 CHANNELS COMPETITION/Striatum D2/Striatum D2  ==
  Channel : Inport
  Band-Limited White Noise : simulink/Sources/Band-Limited White Noise  Cov=[0]  Ts=0.1  seed=[23341]
  Demux : Demux  Outputs=5
  Mux : Mux  Inputs=5
  Scope : Scope
  StrSat : Subsystem
  StrSat1 : Subsystem
  StrSat2 : Subsystem
  StrSat3 : Subsystem
  StrSat4 : Subsystem
  Sum : Sum
  w_s : Gain  Gain=w_s
  Striatum D1 Out : Outport
  wires:
  Channel/1 -> Sum/1
  Sum/1 -> w_s/1
  Mux/1 -> Striatum D1 Out/1, Scope/1
  Band-Limited White Noise/1 -> Sum/2
  Demux/1 -> StrSat/1(In1)
  StrSat/1(Out1) -> Mux/1
  Demux/2 -> StrSat1/1(In1)
  StrSat1/1(Out1) -> Mux/2
  Demux/3 -> StrSat2/1(In1)
  StrSat2/1(Out1) -> Mux/3
  Demux/4 -> StrSat3/1(In1)
  StrSat3/1(Out1) -> Mux/4
  Demux/5 -> StrSat4/1(In1)
  StrSat4/1(Out1) -> Mux/5
  w_s/1 -> Demux/1

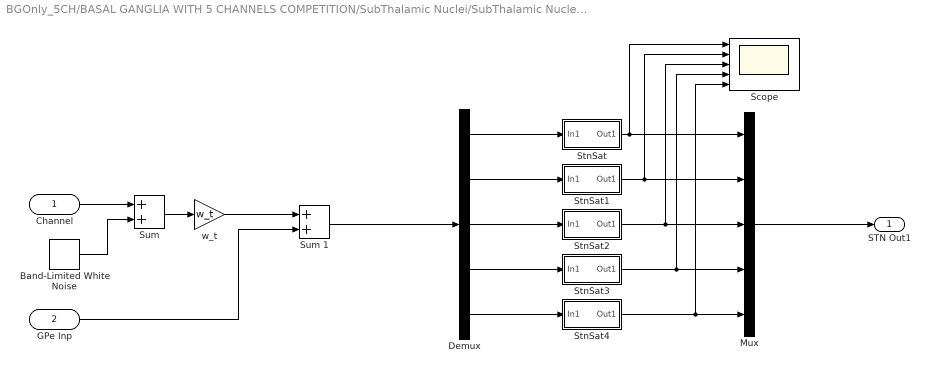
== system BGOnly_5CH/BASAL GANGLIA WITH 5 CHANNELS COMPETITION/SubThalamic Nuclei/SubThalamic Nucleus (STN)  ==
  Channel : Inport
  GPe Inp : Inport  Port=2
  Band-Limited White Noise : simulink/Sources/Band-Limited White Noise  Cov=[0]  Ts=0.1  seed=[23341]
  Demux : Demux  Outputs=5
  Mux : Mux  Inputs=5
  Scope : Scope  NumInputPorts=5
  StnSat : Subsystem
  StnSat1 : Subsystem
  StnSat2 : Subsystem
  StnSat3 : Subsystem
  StnSat4 : Subsystem
  "Sum " : Sum
  Sum 1 : Sum
  w_t : Gain  Gain=w_t
  STN Out1 : Outport
  wires:
  w_t/1 -> Sum 1/1
  Channel/1 -> "Sum "/1
  Band-Limited White Noise/1 -> "Sum "/2
  "Sum "/1 -> w_t/1
  GPe Inp/1 -> Sum 1/2
  Mux/1 -> STN Out1/1
  Demux/1 -> StnSat/1(In1)
  Demux/2 -> StnSat1/1(In1)
  StnSat1/1(Out1) -> Scope/2, Mux/2
  Demux/3 -> StnSat2/1(In1)
  StnSat2/1(Out1) -> Scope/3, Mux/3
  Demux/4 -> StnSat3/1(In1)
  StnSat3/1(Out1) -> Scope/4, Mux/4
  Demux/5 -> StnSat4/1(In1)
  StnSat4/1(Out1) -> Scope/5, Mux/5
  StnSat/1(Out1) -> Scope/1, Mux/1
  Sum 1/1 -> Demux/1

== system BGOnly_5CH/BASAL GANGLIA WITH 5 CHANNELS COMPETITION/GPe/GPe CH1/GPeSat ==
  In1 : Inport
  "Leaky-Integrator Striatum D1 " : ZeroPole  Zeros=[]  Poles=[-1/teta]  Gain=[1.5/teta]
  Sigmoidal MF : fuzblock/Membership  Functions/Sigmoidal MF  a=alpha_gpe  c=beta_gpe
      settings: SourceProductName=Fuzzy Logic Toolbox  SourceProductBaseCode=FL
  Out1 : Outport
  wires:
  Sigmoidal MF/1 -> Out1/1
  "Leaky-Integrator Striatum D1 "/1 -> Sigmoidal MF/1
  In1/1 -> "Leaky-Integrator Striatum D1 "/1

== system BGOnly_5CH/BASAL GANGLIA WITH 5 CHANNELS COMPETITION/GPe/GPe CH1/GPeSat1 ==
  In1 : Inport
  "Leaky-Integrator Striatum D1 " : ZeroPole  Zeros=[]  Poles=[-1/teta]  Gain=[1.5/teta]
  Sigmoidal MF : fuzblock/Membership  Functions/Sigmoidal MF  a=alpha_gpe  c=beta_gpe
      settings: SourceProductName=Fuzzy Logic Toolbox  SourceProductBaseCode=FL
  Out1 : Outport
  wires:
  Sigmoidal MF/1 -> Out1/1
  "Leaky-Integrator Striatum D1 "/1 -> Sigmoidal MF/1
  In1/1 -> "Leaky-Integrator Striatum D1 "/1

== system BGOnly_5CH/BASAL GANGLIA WITH 5 CHANNELS COMPETITION/GPe/GPe CH1/GPeSat2 ==
  In1 : Inport
  "Leaky-Integrator Striatum D1 " : ZeroPole  Zeros=[]  Poles=[-1/teta]  Gain=[1.5/teta]
  Sigmoidal MF : fuzblock/Membership  Functions/Sigmoidal MF  a=alpha_gpe  c=beta_gpe
      settings: SourceProductName=Fuzzy Logic Toolbox  SourceProductBaseCode=FL
  Out1 : Outport
  wires:
  Sigmoidal MF/1 -> Out1/1
  "Leaky-Integrator Striatum D1 "/1 -> Sigmoidal MF/1
  In1/1 -> "Leaky-Integrator Striatum D1 "/1

== system BGOnly_5CH/BASAL GANGLIA WITH 5 CHANNELS COMPETITION/GPe/GPe CH1/GPeSat3 ==
  In1 : Inport
  "Leaky-Integrator Striatum D1 " : ZeroPole  Zeros=[]  Poles=[-1/teta]  Gain=[1.5/teta]
  Sigmoidal MF : fuzblock/Membership  Functions/Sigmoidal MF  a=alpha_gpe  c=beta_gpe
      settings: SourceProductName=Fuzzy Logic Toolbox  SourceProductBaseCode=FL
  Out1 : Outport
  wires:
  Sigmoidal MF/1 -> Out1/1
  "Leaky-Integrator Striatum D1 "/1 -> Sigmoidal MF/1
  In1/1 -> "Leaky-Integrator Striatum D1 "/1

== system BGOnly_5CH/BASAL GANGLIA WITH 5 CHANNELS COMPETITION/GPe/GPe CH1/GPeSat4 ==
  In1 : Inport
  "Leaky-Integrator Striatum D1 " : ZeroPole  Zeros=[]  Poles=[-1/teta]  Gain=[1.5/teta]
  Sigmoidal MF : fuzblock/Membership  Functions/Sigmoidal MF  a=alpha_gpe  c=beta_gpe
      settings: SourceProductName=Fuzzy Logic Toolbox  SourceProductBaseCode=FL
  Out1 : Outport
  wires:
  Sigmoidal MF/1 -> Out1/1
  "Leaky-Integrator Striatum D1 "/1 -> Sigmoidal MF/1
  In1/1 -> "Leaky-Integrator Striatum D1 "/1

== system BGOnly_5CH/BASAL GANGLIA WITH 5 CHANNELS COMPETITION/GPi/GPinternal/GPinternal ==
  In1 : Inport
  "Leaky-Integrator Striatum D1 " : ZeroPole  Zeros=[]  Poles=[-1/teta]  Gain=[1.5/teta]
  Sigmoidal MF : fuzblock/Membership  Functions/Sigmoidal MF  a=alpha_gpi  c=beta_gpi
      settings: SourceProductName=Fuzzy Logic Toolbox  SourceProductBaseCode=FL
  Out1 : Outport
  wires:
  Sigmoidal MF/1 -> Out1/1
  "Leaky-Integrator Striatum D1 "/1 -> Sigmoidal MF/1
  In1/1 -> "Leaky-Integrator Striatum D1 "/1

== system BGOnly_5CH/BASAL GANGLIA WITH 5 CHANNELS COMPETITION/GPi/GPinternal/GPinternal1 ==
  In1 : Inport
  "Leaky-Integrator Striatum D1 " : ZeroPole  Zeros=[]  Poles=[-1/teta]  Gain=[1.5/teta]
  Sigmoidal MF : fuzblock/Membership  Functions/Sigmoidal MF  a=alpha_gpi  c=beta_gpi
      settings: SourceProductName=Fuzzy Logic Toolbox  SourceProductBaseCode=FL
  Out1 : Outport
  wires:
  Sigmoidal MF/1 -> Out1/1
  "Leaky-Integrator Striatum D1 "/1 -> Sigmoidal MF/1
  In1/1 -> "Leaky-Integrator Striatum D1 "/1

== system BGOnly_5CH/BASAL GANGLIA WITH 5 CHANNELS COMPETITION/GPi/GPinternal/GPinternal2 ==
  In1 : Inport
  "Leaky-Integrator Striatum D1 " : ZeroPole  Zeros=[]  Poles=[-1/teta]  Gain=[1.5/teta]
  Sigmoidal MF : fuzblock/Membership  Functions/Sigmoidal MF  a=alpha_gpi  c=beta_gpi
      settings: SourceProductName=Fuzzy Logic Toolbox  SourceProductBaseCode=FL
  Out1 : Outport
  wires:
  Sigmoidal MF/1 -> Out1/1
  "Leaky-Integrator Striatum D1 "/1 -> Sigmoidal MF/1
  In1/1 -> "Leaky-Integrator Striatum D1 "/1

== system BGOnly_5CH/BASAL GANGLIA WITH 5 CHANNELS COMPETITION/GPi/GPinternal/GPinternal3 ==
  In1 : Inport
  "Leaky-Integrator Striatum D1 " : ZeroPole  Zeros=[]  Poles=[-1/teta]  Gain=[1.5/teta]
  Sigmoidal MF : fuzblock/Membership  Functions/Sigmoidal MF  a=alpha_gpi  c=beta_gpi
      settings: SourceProductName=Fuzzy Logic Toolbox  SourceProductBaseCode=FL
  Out1 : Outport
  wires:
  Sigmoidal MF/1 -> Out1/1
  "Leaky-Integrator Striatum D1 "/1 -> Sigmoidal MF/1
  In1/1 -> "Leaky-Integrator Striatum D1 "/1

== system BGOnly_5CH/BASAL GANGLIA WITH 5 CHANNELS COMPETITION/GPi/GPinternal/GPinternal4 ==
  In1 : Inport
  "Leaky-Integrator Striatum D1 " : ZeroPole  Zeros=[]  Poles=[-1/teta]  Gain=[1.5/teta]
  Sigmoidal MF : fuzblock/Membership  Functions/Sigmoidal MF  a=alpha_gpi  c=beta_gpi
      settings: SourceProductName=Fuzzy Logic Toolbox  SourceProductBaseCode=FL
  Out1 : Outport
  wires:
  Sigmoidal MF/1 -> Out1/1
  "Leaky-Integrator Striatum D1 "/1 -> Sigmoidal MF/1
  In1/1 -> "Leaky-Integrator Striatum D1 "/1

== system BGOnly_5CH/BASAL GANGLIA WITH 5 CHANNELS COMPETITION/Striatum D1 /Striatum D1 /StrSat ==
  In1 : Inport
  "Leaky-Integrator Striatum D1 " : ZeroPole  Zeros=[]  Poles=[-1/teta]  Gain=[1.5/teta]
  Sigmoidal MF : fuzblock/Membership  Functions/Sigmoidal MF  a=alpha_str  c=beta_str
      settings: SourceProductName=Fuzzy Logic Toolbox  SourceProductBaseCode=FL
  Out1 : Outport
  wires:
  Sigmoidal MF/1 -> Out1/1
  "Leaky-Integrator Striatum D1 "/1 -> Sigmoidal MF/1
  In1/1 -> "Leaky-Integrator Striatum D1 "/1

== system BGOnly_5CH/BASAL GANGLIA WITH 5 CHANNELS COMPETITION/Striatum D1 /Striatum D1 /StrSat1 ==
  In1 : Inport
  "Leaky-Integrator Striatum D1 " : ZeroPole  Zeros=[]  Poles=[-1/teta]  Gain=[1.5/teta]
  Sigmoidal MF : fuzblock/Membership  Functions/Sigmoidal MF  a=alpha_str  c=beta_str
      settings: SourceProductName=Fuzzy Logic Toolbox  SourceProductBaseCode=FL
  Out1 : Outport
  wires:
  Sigmoidal MF/1 -> Out1/1
  "Leaky-Integrator Striatum D1 "/1 -> Sigmoidal MF/1
  In1/1 -> "Leaky-Integrator Striatum D1 "/1

== system BGOnly_5CH/BASAL GANGLIA WITH 5 CHANNELS COMPETITION/Striatum D1 /Striatum D1 /StrSat2 ==
  In1 : Inport
  "Leaky-Integrator Striatum D1 " : ZeroPole  Zeros=[]  Poles=[-1/teta]  Gain=[1.5/teta]
  Sigmoidal MF : fuzblock/Membership  Functions/Sigmoidal MF  a=alpha_str  c=beta_str
      settings: SourceProductName=Fuzzy Logic Toolbox  SourceProductBaseCode=FL
  Out1 : Outport
  wires:
  Sigmoidal MF/1 -> Out1/1
  "Leaky-Integrator Striatum D1 "/1 -> Sigmoidal MF/1
  In1/1 -> "Leaky-Integrator Striatum D1 "/1

== system BGOnly_5CH/BASAL GANGLIA WITH 5 CHANNELS COMPETITION/Striatum D1 /Striatum D1 /StrSat3 ==
  In1 : Inport
  "Leaky-Integrator Striatum D1 " : ZeroPole  Zeros=[]  Poles=[-1/teta]  Gain=[1.5/teta]
  Sigmoidal MF : fuzblock/Membership  Functions/Sigmoidal MF  a=alpha_str  c=beta_str
      settings: SourceProductName=Fuzzy Logic Toolbox  SourceProductBaseCode=FL
  Out1 : Outport
  wires:
  Sigmoidal MF/1 -> Out1/1
  "Leaky-Integrator Striatum D1 "/1 -> Sigmoidal MF/1
  In1/1 -> "Leaky-Integrator Striatum D1 "/1

== system BGOnly_5CH/BASAL GANGLIA WITH 5 CHANNELS COMPETITION/Striatum D1 /Striatum D1 /StrSat4 ==
  In1 : Inport
  "Leaky-Integrator Striatum D1 " : ZeroPole  Zeros=[]  Poles=[-1/teta]  Gain=[1.5/teta]
  Sigmoidal MF : fuzblock/Membership  Functions/Sigmoidal MF  a=alpha_str  c=beta_str
      settings: SourceProductName=Fuzzy Logic Toolbox  SourceProductBaseCode=FL
  Out1 : Outport
  wires:
  Sigmoidal MF/1 -> Out1/1
  "Leaky-Integrator Striatum D1 "/1 -> Sigmoidal MF/1
  In1/1 -> "Leaky-Integrator Striatum D1 "/1

== system BGOnly_5CH/BASAL GANGLIA WITH 5 CHANNELS COMPETITION/Striatum D2/Striatum D2 /StrSat ==
  In1 : Inport
  "Leaky-Integrator Striatum D1 " : ZeroPole  Zeros=[]  Poles=[-1/teta]  Gain=[1.5/teta]
  Sigmoidal MF : fuzblock/Membership  Functions/Sigmoidal MF  a=alpha_str  c=beta_str
      settings: SourceProductName=Fuzzy Logic Toolbox  SourceProductBaseCode=FL
  Out1 : Outport
  wires:
  Sigmoidal MF/1 -> Out1/1
  "Leaky-Integrator Striatum D1 "/1 -> Sigmoidal MF/1
  In1/1 -> "Leaky-Integrator Striatum D1 "/1

== system BGOnly_5CH/BASAL GANGLIA WITH 5 CHANNELS COMPETITION/Striatum D2/Striatum D2 /StrSat1 ==
  In1 : Inport
  "Leaky-Integrator Striatum D1 " : ZeroPole  Zeros=[]  Poles=[-1/teta]  Gain=[1.5/teta]
  Sigmoidal MF : fuzblock/Membership  Functions/Sigmoidal MF  a=alpha_str  c=beta_str
      settings: SourceProductName=Fuzzy Logic Toolbox  SourceProductBaseCode=FL
  Out1 : Outport
  wires:
  Sigmoidal MF/1 -> Out1/1
  "Leaky-Integrator Striatum D1 "/1 -> Sigmoidal MF/1
  In1/1 -> "Leaky-Integrator Striatum D1 "/1

== system BGOnly_5CH/BASAL GANGLIA WITH 5 CHANNELS COMPETITION/Striatum D2/Striatum D2 /StrSat2 ==
  In1 : Inport
  "Leaky-Integrator Striatum D1 " : ZeroPole  Zeros=[]  Poles=[-1/teta]  Gain=[1.5/teta]
  Sigmoidal MF : fuzblock/Membership  Functions/Sigmoidal MF  a=alpha_str  c=beta_str
      settings: SourceProductName=Fuzzy Logic Toolbox  SourceProductBaseCode=FL
  Out1 : Outport
  wires:
  Sigmoidal MF/1 -> Out1/1
  "Leaky-Integrator Striatum D1 "/1 -> Sigmoidal MF/1
  In1/1 -> "Leaky-Integrator Striatum D1 "/1

== system BGOnly_5CH/BASAL GANGLIA WITH 5 CHANNELS COMPETITION/Striatum D2/Striatum D2 /StrSat3 ==
  In1 : Inport
  "Leaky-Integrator Striatum D1 " : ZeroPole  Zeros=[]  Poles=[-1/teta]  Gain=[1.5/teta]
  Sigmoidal MF : fuzblock/Membership  Functions/Sigmoidal MF  a=alpha_str  c=beta_str
      settings: SourceProductName=Fuzzy Logic Toolbox  SourceProductBaseCode=FL
  Out1 : Outport
  wires:
  Sigmoidal MF/1 -> Out1/1
  "Leaky-Integrator Striatum D1 "/1 -> Sigmoidal MF/1
  In1/1 -> "Leaky-Integrator Striatum D1 "/1

== system BGOnly_5CH/BASAL GANGLIA WITH 5 CHANNELS COMPETITION/Striatum D2/Striatum D2 /StrSat4 ==
  In1 : Inport
  "Leaky-Integrator Striatum D1 " : ZeroPole  Zeros=[]  Poles=[-1/teta]  Gain=[1.5/teta]
  Sigmoidal MF : fuzblock/Membership  Functions/Sigmoidal MF  a=alpha_str  c=beta_str
      settings: SourceProductName=Fuzzy Logic Toolbox  SourceProductBaseCode=FL
  Out1 : Outport
  wires:
  Sigmoidal MF/1 -> Out1/1
  "Leaky-Integrator Striatum D1 "/1 -> Sigmoidal MF/1
  In1/1 -> "Leaky-Integrator Striatum D1 "/1

== system BGOnly_5CH/BASAL GANGLIA WITH 5 CHANNELS COMPETITION/SubThalamic Nuclei/SubThalamic Nucleus (STN) /StnSat ==
  In1 : Inport
  "Leaky-Integrator Striatum D1 " : ZeroPole  Zeros=[]  Poles=[-1/teta]  Gain=[1.5/teta]
  Sigmoidal MF : fuzblock/Membership  Functions/Sigmoidal MF  a=alpha_stn  c=beta_stn
      settings: SourceProductName=Fuzzy Logic Toolbox  SourceProductBaseCode=FL
  Out1 : Outport
  wires:
  Sigmoidal MF/1 -> Out1/1
  "Leaky-Integrator Striatum D1 "/1 -> Sigmoidal MF/1
  In1/1 -> "Leaky-Integrator Striatum D1 "/1

== system BGOnly_5CH/BASAL GANGLIA WITH 5 CHANNELS COMPETITION/SubThalamic Nuclei/SubThalamic Nucleus (STN) /StnSat1 ==
  In1 : Inport
  "Leaky-Integrator Striatum D1 " : ZeroPole  Zeros=[]  Poles=[-1/teta]  Gain=[1.5/teta]
  Sigmoidal MF : fuzblock/Membership  Functions/Sigmoidal MF  a=alpha_stn  c=beta_stn
      settings: SourceProductName=Fuzzy Logic Toolbox  SourceProductBaseCode=FL
  Out1 : Outport
  wires:
  Sigmoidal MF/1 -> Out1/1
  "Leaky-Integrator Striatum D1 "/1 -> Sigmoidal MF/1
  In1/1 -> "Leaky-Integrator Striatum D1 "/1

== system BGOnly_5CH/BASAL GANGLIA WITH 5 CHANNELS COMPETITION/SubThalamic Nuclei/SubThalamic Nucleus (STN) /StnSat2 ==
  In1 : Inport
  "Leaky-Integrator Striatum D1 " : ZeroPole  Zeros=[]  Poles=[-1/teta]  Gain=[1.5/teta]
  Sigmoidal MF : fuzblock/Membership  Functions/Sigmoidal MF  a=alpha_stn  c=beta_stn
      settings: SourceProductName=Fuzzy Logic Toolbox  SourceProductBaseCode=FL
  Out1 : Outport
  wires:
  Sigmoidal MF/1 -> Out1/1
  "Leaky-Integrator Striatum D1 "/1 -> Sigmoidal MF/1
  In1/1 -> "Leaky-Integrator Striatum D1 "/1

== system BGOnly_5CH/BASAL GANGLIA WITH 5 CHANNELS COMPETITION/SubThalamic Nuclei/SubThalamic Nucleus (STN) /StnSat3 ==
  In1 : Inport
  "Leaky-Integrator Striatum D1 " : ZeroPole  Zeros=[]  Poles=[-1/teta]  Gain=[1.5/teta]
  Sigmoidal MF : fuzblock/Membership  Functions/Sigmoidal MF  a=alpha_stn  c=beta_stn
      settings: SourceProductName=Fuzzy Logic Toolbox  SourceProductBaseCode=FL
  Out1 : Outport
  wires:
  Sigmoidal MF/1 -> Out1/1
  "Leaky-Integrator Striatum D1 "/1 -> Sigmoidal MF/1
  In1/1 -> "Leaky-Integrator Striatum D1 "/1

== system BGOnly_5CH/BASAL GANGLIA WITH 5 CHANNELS COMPETITION/SubThalamic Nuclei/SubThalamic Nucleus (STN) /StnSat4 ==
  In1 : Inport
  "Leaky-Integrator Striatum D1 " : ZeroPole  Zeros=[]  Poles=[-1/teta]  Gain=[1.5/teta]
  Sigmoidal MF : fuzblock/Membership  Functions/Sigmoidal MF  a=alpha_stn  c=beta_stn
      settings: SourceProductName=Fuzzy Logic Toolbox  SourceProductBaseCode=FL
  Out1 : Outport
  wires:
  Sigmoidal MF/1 -> Out1/1
  "Leaky-Integrator Striatum D1 "/1 -> Sigmoidal MF/1
  In1/1 -> "Leaky-Integrator Striatum D1 "/1
